simulink model "adder"  (R2017a)
settings: Solver=VariableStepAuto  StartTime=0.0  StopTime=10.0  RelTol=1e-3
settings Model: Creator=Pc  LastModifiedBy=Pc

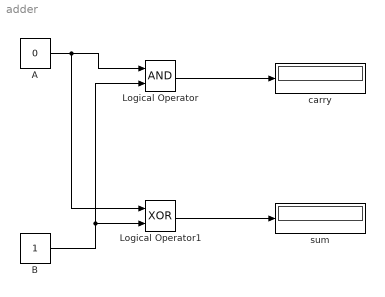
== system adder ==
  A : Constant  Value=0  OutDataTypeStr=boolean
  B : Constant  OutDataTypeStr=boolean
  Logical Operator : Logic  AllPortsSameDT=off  OutDataTypeStr=boolean
  Logical Operator1 : Logic  Operator=XOR  AllPortsSameDT=off  OutDataTypeStr=boolean
  carry : Display
  sum : Display
  wires:
  A/1 -> Logical Operator1/1, Logical Operator/1
  B/1 -> Logical Operator1/2, Logical Operator/2
  Logical Operator/1 -> carry/1
  Logical Operator1/1 -> sum/1
